simulink model "simulink_s2_22b_22c_2020a_03"  (R2020a)
settings: Solver=VariableStepAuto  StartTime=0.0  StopTime=10.0  RelTol=1e-3
settings Model: Creator=Admin  LastModifiedBy=Admin
settings DebuggingCC: UnconnectedInputMsg=none  UnconnectedOutputMsg=none  UnconnectedLineMsg=none  SFMachineParentedDataDiag=error
settings ModelReferenceCC: EnableRefExpFcnMdlSchedulingChecks=off
settings RTWCC: Description=Generic Real-Time Target

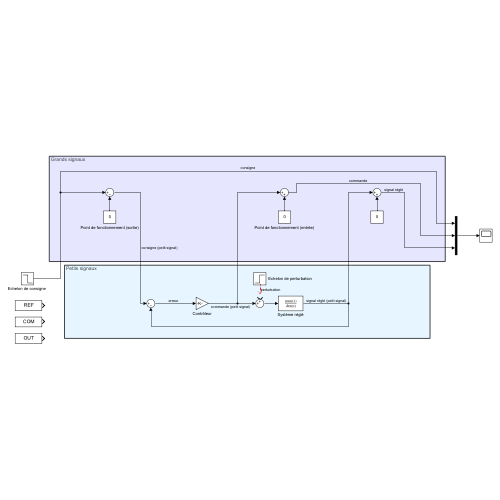
[thumbnail: Simulink's stored preview of the top-level diagram]
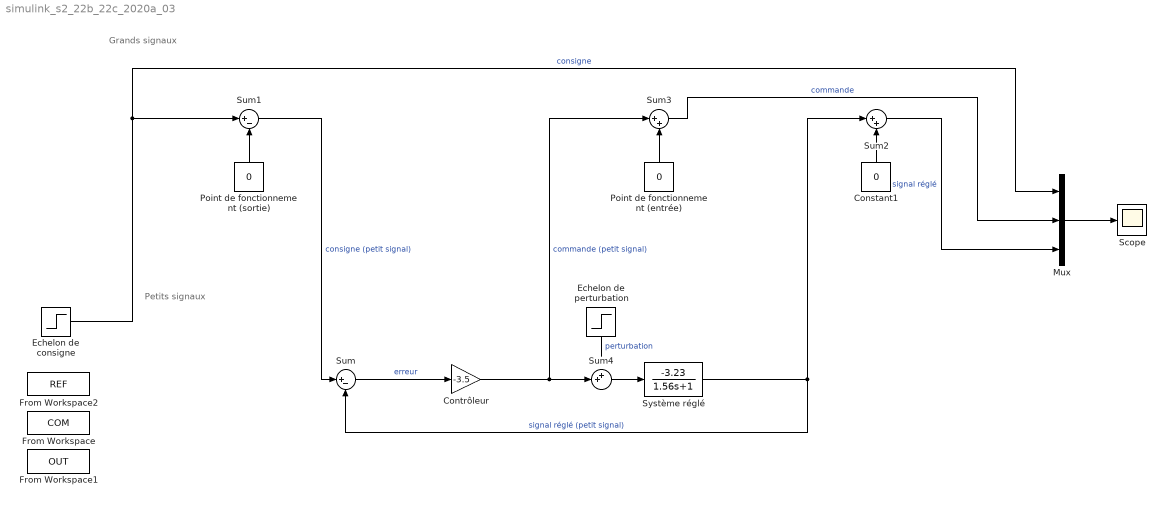
== system simulink_s2_22b_22c_2020a_03 ==
  note: Petits signaux
  note: Grands signaux
  Constant1 : Constant  Value=0
  Contrôleur : Gain  Gain=-3.5
  "Echelon de consigne " : Step  Before=-4.67  After=-8  SampleTime=0
  Echelon de perturbation : Step  After=0.5  SampleTime=0
  From Workspace : FromWorkspace  VariableName=COM
  From Workspace1 : FromWorkspace  VariableName=OUT
  From Workspace2 : FromWorkspace  VariableName=REF
  Mux : Mux  Inputs=3
  Point de fonctionnement (entrée) : Constant  Value=0
  Point de fonctionnement (sortie) : Constant  Value=0
  Scope : Scope
  Sum : Sum  Inputs=|+-
  Sum1 : Sum  Inputs=|+-
  Sum2 : Sum  Inputs=|++
  Sum3 : Sum  Inputs=|++
  Sum4 : Sum  Inputs=++|
  Système réglé : TransferFcn  Numerator=[-3.23]  Denominator=[1.56 1]
  wires:
  Sum/1 -> Contrôleur/1  "erreur"
  Contrôleur/1 -> Sum4/2, Sum3/1  "commande (petit signal)"
  Système réglé/1 -> Sum2/1, Sum/2  "signal réglé (petit signal)"
  Constant1/1 -> Sum2/2
  Mux/1 -> Scope/1
  Sum2/1 -> Mux/3  "signal réglé"
  "Echelon de consigne "/1 -> Sum1/1, Mux/1  "consigne"
  Sum1/1 -> Sum/1  "consigne (petit signal)"
  Point de fonctionnement (sortie)/1 -> Sum1/2
  Point de fonctionnement (entrée)/1 -> Sum3/2
  Sum3/1 -> Mux/2  "commande"
  Sum4/1 -> Système réglé/1
  Echelon de perturbation/1 -> ?  "perturbation"
